simulink model "MEMS_Gyro_Structure_Model_231114_tb"  (R2022b)
settings: Solver=VariableStepAuto  StartTime=0.0  StopTime=3  MaxStep=1e-5  RelTol=1e-3
libraries: cstblocks x1
settings Model: Creator=admin  LastModifiedBy=admin

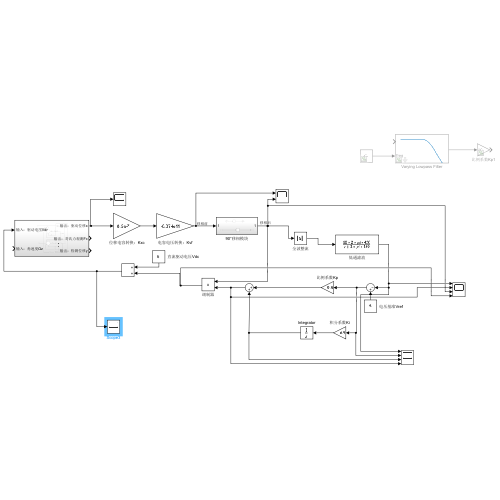
[thumbnail: Simulink's stored preview of the top-level diagram]
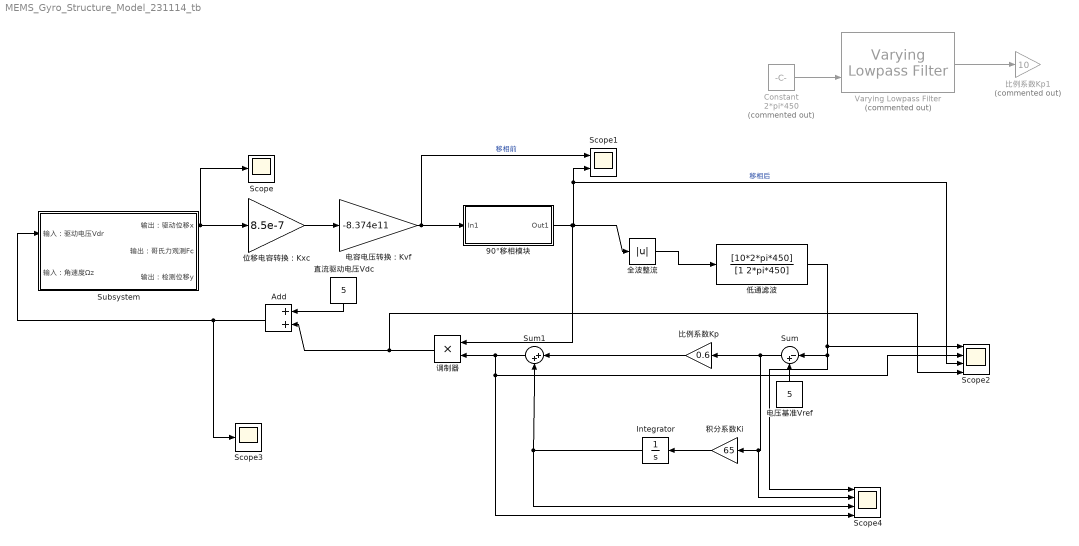
== system MEMS_Gyro_Structure_Model_231114_tb ==
  90°移相模块 : Subsystem
  Add : Sum
  Constant : Constant  Commented=on  Value=2*pi*450
  Integrator : Integrator
  Scope : Scope
  Scope1 : Scope  NumInputPorts=2
  Scope2 : Scope  NumInputPorts=4
  Scope3 : Scope
  Scope4 : Scope  NumInputPorts=4
  Subsystem : Subsystem
  Sum : Sum  Inputs=|-+
  Sum1 : Sum  Inputs=|++
  Varying Lowpass Filter : cstblocks/Linear Parameter Varying/Varying Lowpass Filter  Commented=on  N=1
  位移电容转换：Kxc : Gain  Gain=8.5e-7
  低通滤波 : TransferFcn  Numerator=[10*2*pi*450]  Denominator=[1 2*pi*450]
  全波整流 : Abs  SaturateOnIntegerOverflow=off
  比例系数Kp : Gain  Gain=0.6
  比例系数Kp1 : Gain  Commented=on  Gain=10
  电压基准Vref : Constant  Value=5
  电容电压转换：Kvf : Gain  Gain=-8.374e11
  直流驱动电压Vdc : Constant  Value=5
  积分系数Ki : Gain  Gain=65
  调制器 : Product
  wires:
  Add/1 -> Scope3/1, Subsystem/1(输入：驱动电压Vdr)
  Subsystem/1(输出：驱动位移x) -> Scope/1, 位移电容转换：Kxc/1
  90°移相模块/1(Out1) -> 全波整流/1, Scope2/3, Scope1/2, 调制器/1  "移相后"
  位移电容转换：Kxc/1 -> 电容电压转换：Kvf/1
  电容电压转换：Kvf/1 -> Scope1/1, 90°移相模块/1(In1)  "移相前"
  Sum1/1 -> Scope4/4, Scope2/2, 调制器/2
  直流驱动电压Vdc/1 -> Add/1
  调制器/1 -> Scope2/4, Add/2
  全波整流/1 -> 低通滤波/1
  比例系数Kp/1 -> Sum1/1
  电压基准Vref/1 -> Sum/2
  Sum/1 -> 比例系数Kp/1, Scope4/2, 积分系数Ki/1
  Integrator/1 -> Scope4/3, Sum1/2
  积分系数Ki/1 -> Integrator/1
  Constant/1 -> Varying Lowpass Filter/2
  Varying Lowpass Filter/1 -> 比例系数Kp1/1
  低通滤波/1 -> Scope4/1, Sum/1, Scope2/1

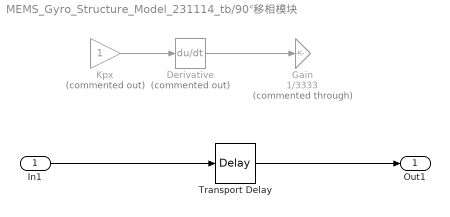
== system MEMS_Gyro_Structure_Model_231114_tb/90°移相模块 ==
  In1 : Inport
  Derivative : Derivative  Commented=on
  Gain : Gain  Commented=through  Gain=1/3333
  Kpx : Gain  Commented=on
  Transport Delay : TransportDelay  DelayTime=1/(3489.44*4)
  Out1 : Outport
  wires:
  In1/1 -> Transport Delay/1
  Transport Delay/1 -> Out1/1
  Derivative/1 -> Gain/1
  Kpx/1 -> Derivative/1

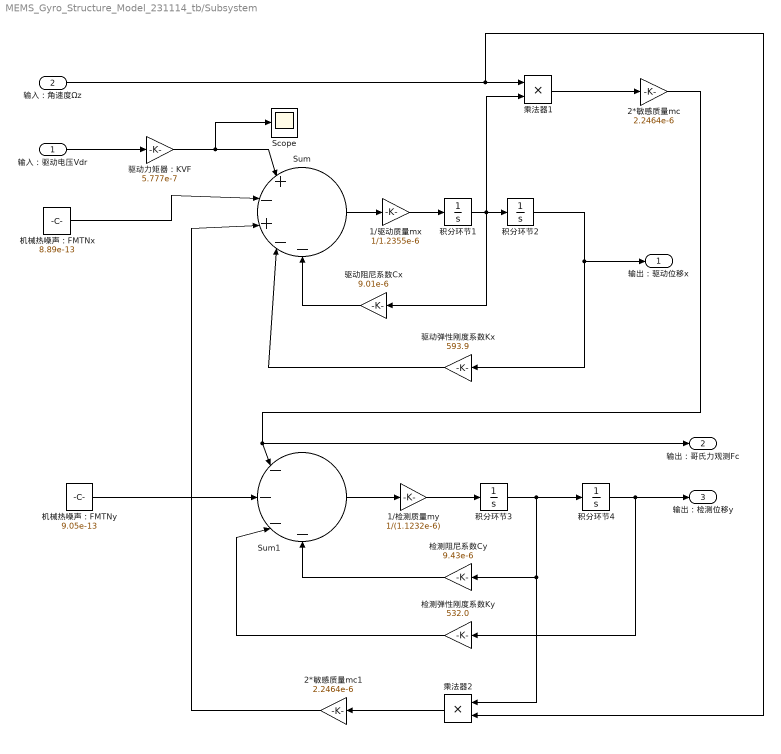
== system MEMS_Gyro_Structure_Model_231114_tb/Subsystem ==
  输入：驱动电压Vdr : Inport
  输入：角速度Ωz : Inport  Port=2
  1/检测质量my : Gain  Gain=1/(1.1232e-6)
  1/驱动质量mx : Gain  Gain=1/1.2355e-6
  2*敏感质量mc : Gain  Gain=2.2464e-6
  2*敏感质量mc1 : Gain  Gain=2.2464e-6
  Scope : Scope
  Sum : Sum  Inputs=|+-+--
  Sum1 : Sum  Inputs=|----
  乘法器1 : Product
  乘法器2 : Product
  机械热噪声：FMTNx : Constant  Value=8.89e-13
  机械热噪声：FMTNy : Constant  Value=9.05e-13
  检测弹性刚度系数Ky : Gain  Gain=532.0
  检测阻尼系数Cy : Gain  Gain=9.43e-6
  积分环节{1..4} (4 alike) : Integrator
  驱动力矩器：KVF : Gain  Gain=5.777e-7
  驱动弹性刚度系数Kx : Gain  Gain=593.9
  驱动阻尼系数Cx : Gain  Gain=9.01e-6
  输出：驱动位移x : Outport
  输出：哥氏力观测Fc : Outport  Port=2
  输出：检测位移y : Outport  Port=3
  wires:
  1/检测质量my/1 -> 积分环节3/1
  积分环节1/1 -> 驱动阻尼系数Cx/1, 乘法器1/2, 积分环节2/1
  积分环节4/1 -> 输出：检测位移y/1, 检测弹性刚度系数Ky/1
  机械热噪声：FMTNx/1 -> Sum/2
  2*敏感质量mc/1 -> 输出：哥氏力观测Fc/1, Sum1/1
  积分环节3/1 -> 乘法器2/1, 检测阻尼系数Cy/1, 积分环节4/1
  检测弹性刚度系数Ky/1 -> Sum1/3
  Sum1/1 -> 1/检测质量my/1
  输入：驱动电压Vdr/1 -> 驱动力矩器：KVF/1
  机械热噪声：FMTNy/1 -> Sum1/2
  积分环节2/1 -> 输出：驱动位移x/1, 驱动弹性刚度系数Kx/1
  输入：角速度Ωz/1 -> 乘法器2/2, 乘法器1/1
  Sum/1 -> 1/驱动质量mx/1
  驱动阻尼系数Cx/1 -> Sum/5
  2*敏感质量mc1/1 -> Sum/3
  驱动弹性刚度系数Kx/1 -> Sum/4
  乘法器1/1 -> 2*敏感质量mc/1
  驱动力矩器：KVF/1 -> Scope/1, Sum/1
  1/驱动质量mx/1 -> 积分环节1/1
  乘法器2/1 -> 2*敏感质量mc1/1
  检测阻尼系数Cy/1 -> Sum1/4
